simulink model "prob1"  (R2020b)
settings: Solver=VariableStepAuto  StartTime=0.0  StopTime=100  MaxStep=0.001  RelTol=1e-3
model workspace (MAT data in the model file):
  b = Simulink.Parameter
  b.Value = 50
  b.DataType = 'auto'
  b.Dimensions = [1 1]
  k1 = Simulink.Parameter
  k1.Value = 50
  k1.DataType = 'auto'
  k1.Dimensions = [1 1]
  m1 = Simulink.Parameter
  m1.Value = 100
  m1.DataType = 'auto'
  m1.Dimensions = [1 1]
values from neighbouring files (symbols this model uses):
  b = 50    [data.m]
  k1 = 50    [data.m]
  m1 = 100    [data.m]
settings Model: Creator=deves  LastModifiedBy=deves

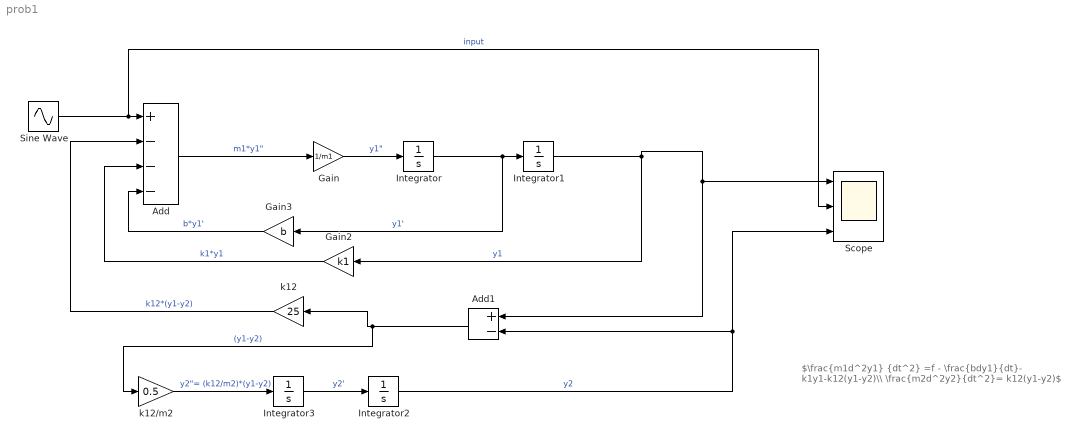
== system prob1 ==
  note: $\frac{m1d^2y1} {dt^2} =f - \frac{bdy1}{dt}- k1y1-k12(y1-y2)\\ \frac{m2d^2y2}{dt^2}= k12(y1-y2)$
  Add : Sum  Inputs=+---
  Add1 : Sum  Inputs=+-
  Gain : Gain  Gain=1/m1
  Gain2 : Gain  Gain=k1
  Gain3 : Gain  Gain=b
  Integrator{,1..3} (4 alike) : Integrator
  Scope : Scope  NumInputPorts=3
  Sine Wave : Sin  Amplitude=2  Frequency=10  SampleTime=0
  k12 : Gain  Gain=25
  k12/m2 : Gain  Gain=0.5
  wires:
  Sine Wave/1 -> Scope/2, Add/1  "input"
  Add/1 -> Gain/1  "m1*y1\""
  Gain/1 -> Integrator/1  "y1\""
  Integrator/1 -> Gain3/1, Integrator1/1  "y1'"
  Integrator3/1 -> Integrator2/1  "y2'"
  Integrator1/1 -> Add1/1, Scope/1, Gain2/1  "y1"
  Integrator2/1 -> Add1/2, Scope/3  "y2"
  Gain3/1 -> Add/4  "b*y1'"
  Gain2/1 -> Add/3  "k1*y1"
  k12/1 -> Add/2  "k12*(y1-y2)"
  k12/m2/1 -> Integrator3/1  "y2\"= (k12/m2)*(y1-y2)"
  Add1/1 -> k12/m2/1, k12/1  "(y1-y2)"
